simulink model "qp_alloc_demo"  (Simulink 8.0)
settings: Solver=ode45  StartTime=0.0  StopTime=10.0  RelTol=1e-3
libraries: qcatlib x1
settings Model: Creator=ola  LastModifiedBy=David  ExtModeAutoUpdateStatusClock=off
settings DataIOCC: SignalLoggingSaveFormat=ModelDataLogs  SignalLoggingName=sigsOut
settings OptimizationCC: BooleanDataType=off
settings DebuggingCC: SaveWithParameterizedLinksMsg=none  SignalResolutionControl=TryResolveAllWithWarning  SolverPrmCheckMsg=none  MultiTaskDSMMsg=warning  MultiTaskCondExecSysMsg=none  StrictBusMsg=None
settings HardwareCC: TargetUnknown=on
settings RTWCC: IncludeERTFirstTime=on
settings GRTTargetCC: CombineOutputUpdateFcns=off  GRTInterface=on

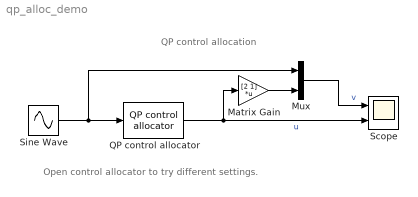
== system qp_alloc_demo ==
  note: QP control allocation
  note: Open control allocator to try different settings.
  Matrix Gain : Gain  Gain=[2 1]  Multiplication=Matrix(K*u)  SaturateOnIntegerOverflow=on  OutDataTypeStr=Inherit: Same as input  ParamDataTypeStr=Inherit: Same as input
  Mux : Mux  Inputs=2
  QP control allocator : qcatlib/QP control allocator  B=[2 1]  plim=[-1 1;-1 1]  rlim=[-1 1;-1 1]*2  T=.1  Wv=1  Wu=eye(2)  ud=[0 0]'  alg=SLS  imax=100  gam=1e6  tol=1e-4
  Scope : Scope  NumInputPorts=2
      settings: TimeRange=10  YMin=-5~-1.2  YMax=5~1.2
  Sine Wave : Sin  Amplitude=2.8  SampleTime=0
  wires:
  Sine Wave/1 -> QP control allocator/1, Mux/1
  Matrix Gain/1 -> Mux/2
  QP control allocator/1 -> Scope/2, Matrix Gain/1  "u"
  Mux/1 -> Scope/1  "v"
